simulink model "trial_model"  (R2019a)
settings: Solver=VariableStepAuto  StartTime=0.0  StopTime=100  FixedStep=1  RelTol=1e-3
undefined symbols (not defined in the file or in its folder): m
libraries: sldelib x1
settings Model: PauseTimes=23  Creator=Chia Jun Shen  LastModifiedBy=Chia Jun Shen

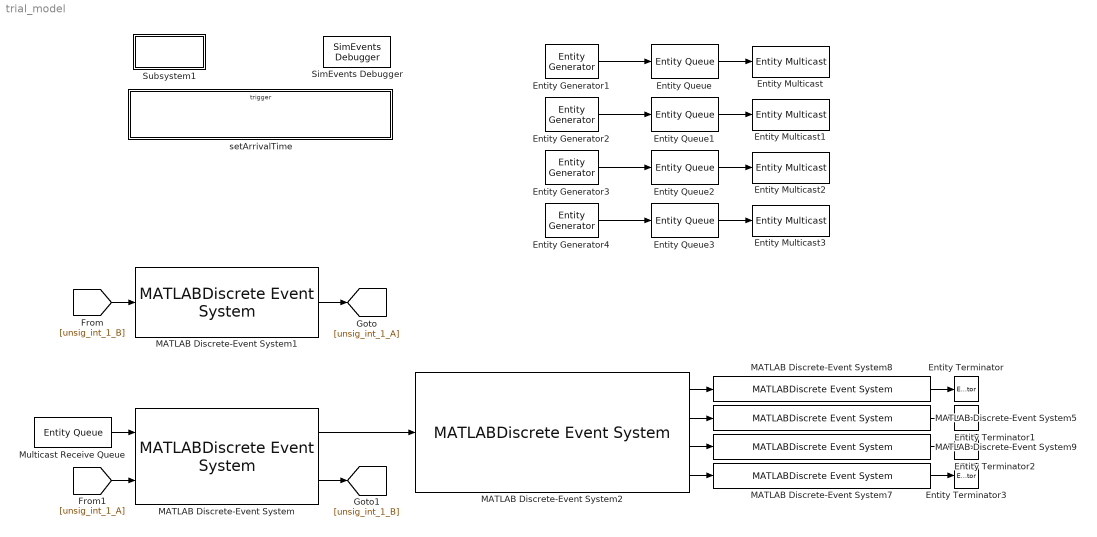
== system trial_model ==
  Entity Generator1 : EntityGenerator  OutputPortMessageModes=m  TimeSource=MATLAB action  IntergenerationTimeAction=|  EntityType=Bus object  EntityTypeName=CAV
      | %mean = 3;
      | %dt = 3 - mean*log(rand());
      | dt = 1000;
  Entity Generator2 : EntityGenerator  OutputPortMessageModes=m  TimeSource=MATLAB action  IntergenerationTimeAction=|  EntityType=Bus object  EntityTypeName=CAV
      | %mean = 3;
      | %dt = 3 - mean*log(rand());
      | dt = 1000;
  Entity Generator3 : EntityGenerator  OutputPortMessageModes=m  TimeSource=MATLAB action  IntergenerationTimeAction=|  EntityType=Bus object  EntityTypeName=CAV
      | %mean = 3;
      | %dt = 3 - mean*log(rand());
      | dt = 1000;
  Entity Generator4 : EntityGenerator  OutputPortMessageModes=m  TimeSource=MATLAB action  IntergenerationTimeAction=|  EntityType=Bus object  EntityTypeName=CAV
      | %mean = 3;
      | %dt = 3 - mean*log(rand());
      | dt = 1000;
  Entity Multicast{,1..3} (4 alike) : EntityMulticast  InputPortMessageModes=m
  Entity Queue : EntityQueue  InputPortMessageModes=m  OutputPortMessageModes=m  Capacity=Inf  EntryAction=|
      | entity.Speed = 15.64;  % average velocity 15.64
      | %entity.Speed = 9 + 2 * rand();
      | entity.Lane = 1;
      | [entity.ArrivalTime,...
      |     entity.ID] = unsig_int_1_setArrivalTime();
      | entity.FinalSpeed = 10;
      | entity.Position = 445;
      | entity.Intersection = 1;
      settings: OutputPortMap=o5
  Entity Queue1 : EntityQueue  InputPortMessageModes=m  OutputPortMessageModes=m  Capacity=Inf  EntryAction=|
      | entity.Speed = 15.64;
      | %entity.Speed = 9 + 2 * rand();
      | entity.Lane = 2;
      | [entity.ArrivalTime,...
      |     entity.ID] = unsig_int_1_setArrivalTime();
      | entity.FinalSpeed = 10;
      | entity.Position = 445;
      | entity.Intersection = 1;
      settings: OutputPortMap=o5
  Entity Queue2 : EntityQueue  InputPortMessageModes=m  OutputPortMessageModes=m  Capacity=Inf  EntryAction=|
      | entity.Speed = 15.64;
      | %entity.Speed = 9 + 2 * rand();
      | entity.Lane = 3;
      | [entity.ArrivalTime,...
      |     entity.ID] = unsig_int_1_setArrivalTime();
      | entity.FinalSpeed = 10;
      | entity.Position = 445;
      | entity.Intersection = 1;
      settings: OutputPortMap=o5
  Entity Queue3 : EntityQueue  InputPortMessageModes=m  OutputPortMessageModes=m  Capacity=Inf  EntryAction=|
      | entity.Speed = 15.64;
      | %entity.Speed = 9 + 2 * rand();
      | entity.Lane = 4;
      | [entity.ArrivalTime,...
      |     entity.ID] = unsig_int_1_setArrivalTime();
      | entity.FinalSpeed = 10;
      | entity.Position = 445;
      | entity.Intersection = 1;
      settings: OutputPortMap=o5
  Entity Terminator{,1..3} (4 alike) : EntityTerminator  InputPortMessageModes=m
  MATLAB Discrete-Event System : MATLABDiscreteEventSystem  InputPortMessageModes=m,m  OutputPortMessageModes=m,m  System=MILP_unsig_int_1_Controller  capacity=100  simulation_step=0.01  MILP_step=4  L=500  d_access=40  S=30  a_acc_max=3  v_max=19  v_ave=15.64  a_dec_max=-4  profiles=repmat( struct( 'speed', @(t) 1, 'position', @(t) 1 ), 1000, 1 )  storageVisited=zeros( 5, 1 )  cavNum=0  arrayMinAccessTime=zeros( 1000, 1 )  arrayLane=zeros( 1000, 1 )  arraySolvedMILP=zeros( 1000, 1 )  run_MILP=0  ready_to_update=0  index=0  delay=0  SimulateUsing=Interpreted execution
      mask Type: MILP_unsig_int_1_Controller
      mask Display:
      | disp(['MILP' char(10) 'CONTROL ZONE']);
      | port_label('input',1,'IN');
      | port_label('input',2,'INFO');
      | port_label('output',1,'OUT');
      | port_label('output',2,'INFO');
  MATLAB Discrete-Event System1 : MATLABDiscreteEventSystem  InputPortMessageModes=m  OutputPortMessageModes=m  System=MILP_unsig_int_1_Coordinator  capacity=100  SimulateUsing=Interpreted execution
      mask Type: MILP_unsig_int_1_Coordinator
      mask Display:
      | disp(['MILP ' char(10) ' COORDINATOR']);
      | port_label('input',1,'IN');
      | port_label('output',1,'OUT');
  MATLAB Discrete-Event System2 : MATLABDiscreteEventSystem  InputPortMessageModes=m  OutputPortMessageModes=m,m,m,m  System=MILP_unsig_int_1_MergingZoneCruiser  capacity=200  simulation_step=0.01  L=400  S=30  d_access=40  storageVisited=0  INT_MAX=2000  SimulateUsing=Interpreted execution
      mask Type: MILP_unsig_int_1_MergingZoneCruiser
      mask Display:
      | disp(['MILP' char(10) 'MERGING ZONE']);
      | port_label('input',1,'CAV');
      | port_label('output',1,'TO WEST');
      | port_label('output',2,'TO SOUTH');
      | port_label('output',3,'TO EAST');
      | port_label('output',4,'TO NORTH');
  MATLAB Discrete-Event System5 : MATLABDiscreteEventSystem  InputPortMessageModes=m  OutputPortMessageModes=m  System=MILP_unsig_int_1_RoadSegment_2  capacity=100  simulation_step=0.01  L=500  d_access=40  S=30  SimulateUsing=Interpreted execution
      mask Type: MILP_unsig_int_1_RoadSegment_2
      mask Display:
      | disp('LEAVE THE INTERSECTION');
      | port_label('input',1,'IN');
      | port_label('output',1,'OUT');
  MATLAB Discrete-Event System7 : MATLABDiscreteEventSystem  InputPortMessageModes=m  OutputPortMessageModes=m  System=MILP_unsig_int_1_RoadSegment_4  capacity=100  simulation_step=0.01  L=500  d_access=40  S=30  SimulateUsing=Interpreted execution
      mask Type: MILP_unsig_int_1_RoadSegment_4
      mask Display:
      | disp('LEAVE THE INTERSECTION');
      | port_label('input',1,'IN');
      | port_label('output',1,'OUT');
  MATLAB Discrete-Event System8 : MATLABDiscreteEventSystem  InputPortMessageModes=m  OutputPortMessageModes=m  System=MILP_unsig_int_1_RoadSegment_1  capacity=100  simulation_step=0.01  L=500  d_access=40  S=30  SimulateUsing=Interpreted execution
      mask Type: MILP_unsig_int_1_RoadSegment_1
      mask Display:
      | disp('LEAVE THE INTERSECTION');
      | port_label('input',1,'IN');
      | port_label('output',1,'OUT');
  MATLAB Discrete-Event System9 : MATLABDiscreteEventSystem  InputPortMessageModes=m  OutputPortMessageModes=m  System=MILP_unsig_int_1_RoadSegment_3  capacity=100  simulation_step=0.01  L=500  d_access=40  S=30  SimulateUsing=Interpreted execution
      mask Type: MILP_unsig_int_1_RoadSegment_3
      mask Display:
      | disp('LEAVE THE INTERSECTION');
      | port_label('input',1,'IN');
      | port_label('output',1,'OUT');
  Multicast Receive Queue : EntityQueue  OutputPortMessageModes=m  Capacity=100  EntityArrivalSource=Multicast
      settings: OutputPortMap=o5
  SimEvents Debugger : sldelib/SimEvents Debugger  EnableDebugger=on  ShowInLibBrowser=0
      settings: SourceProductName=SimEvents  SourceProductBaseCode=SE
  Subsystem1 : Subsystem
      settings: OpenFcn=init_func
      mask Display: disp('init');
  setArrivalTime : Subsystem  TreatAsAtomicUnit=on
  wires:
  Entity Queue1/1 -> Entity Multicast1/1
  Entity Queue/1 -> Entity Multicast/1
  Entity Queue3/1 -> Entity Multicast3/1
  Entity Queue2/1 -> Entity Multicast2/1
  Multicast Receive Queue/1 -> MATLAB Discrete-Event System/1
  MATLAB Discrete-Event System1/1 -> [unsig_int_1_A]
  [unsig_int_1_B] -> MATLAB Discrete-Event System1/1
  [unsig_int_1_A] -> MATLAB Discrete-Event System/2
  MATLAB Discrete-Event System2/1 -> MATLAB Discrete-Event System8/1
  MATLAB Discrete-Event System2/2 -> MATLAB Discrete-Event System5/1
  MATLAB Discrete-Event System2/3 -> MATLAB Discrete-Event System9/1
  MATLAB Discrete-Event System2/4 -> MATLAB Discrete-Event System7/1
  MATLAB Discrete-Event System8/1 -> Entity Terminator/1
  MATLAB Discrete-Event System7/1 -> Entity Terminator3/1
  MATLAB Discrete-Event System9/1 -> Entity Terminator2/1
  MATLAB Discrete-Event System5/1 -> Entity Terminator1/1
  MATLAB Discrete-Event System/1 -> MATLAB Discrete-Event System2/1
  MATLAB Discrete-Event System/2 -> [unsig_int_1_B]
  Entity Generator1/1 -> Entity Queue/1
  Entity Generator2/1 -> Entity Queue1/1
  Entity Generator3/1 -> Entity Queue2/1
  Entity Generator4/1 -> Entity Queue3/1

== system trial_model/Subsystem1 ==

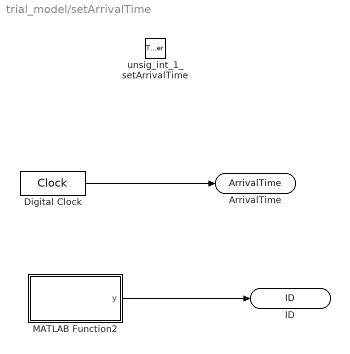
== system trial_model/setArrivalTime ==
  unsig_int_1_setArrivalTime : TriggerPort  TriggerType=function-call  IsSimulinkFunction=on  FunctionName=unsig_int_1_setArrivalTime  FunctionVisibility=scoped  VariantControl=Variant
  Digital Clock : DigitalClock  SampleTime=-1
  MATLAB Function2 : MATLAB Function  TreatAsAtomicUnit=on
  ArrivalTime : ArgOut  DisableCoverage=on  ArgumentName=ArrivalTime
  ID : ArgOut  DisableCoverage=on  Port=2  ArgumentName=ID
  wires:
  Digital Clock/1 -> ArrivalTime/1
  MATLAB Function2/1(y) -> ID/1

== matlab function trial_model/setArrivalTime/MATLAB Function2 ==
  data: y output; unsig_int_1_FF data_store_memory
function y = getID
global unsig_int_1_FF

unsig_int_1_FF = unsig_int_1_FF + 1;
y = unsig_int_1_FF;
